simulink model "modelLiniarizat"  (R2022b)
settings: Solver=VariableStepAuto  StartTime=0.0  StopTime=50.0  RelTol=1e-3
values from neighbouring files (symbols this model uses):
  sys = ss(A_lin, B_lin, C_lin, D_lin)    [NeleptcuDanielAndrei.m]
undefined symbols (not defined in the file or in its folder): par, ustar8, xstar8, ystar8
settings Model: Creator=zuch3e  LastModifiedBy=zuch3e
settings DataIOCC: ReturnWorkspaceOutputs=off

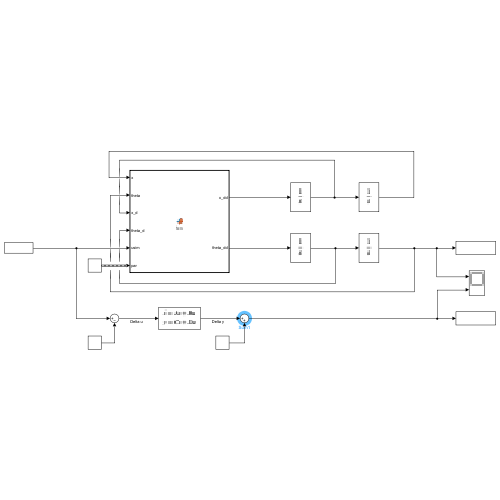
[thumbnail: Simulink's stored preview of the top-level diagram]
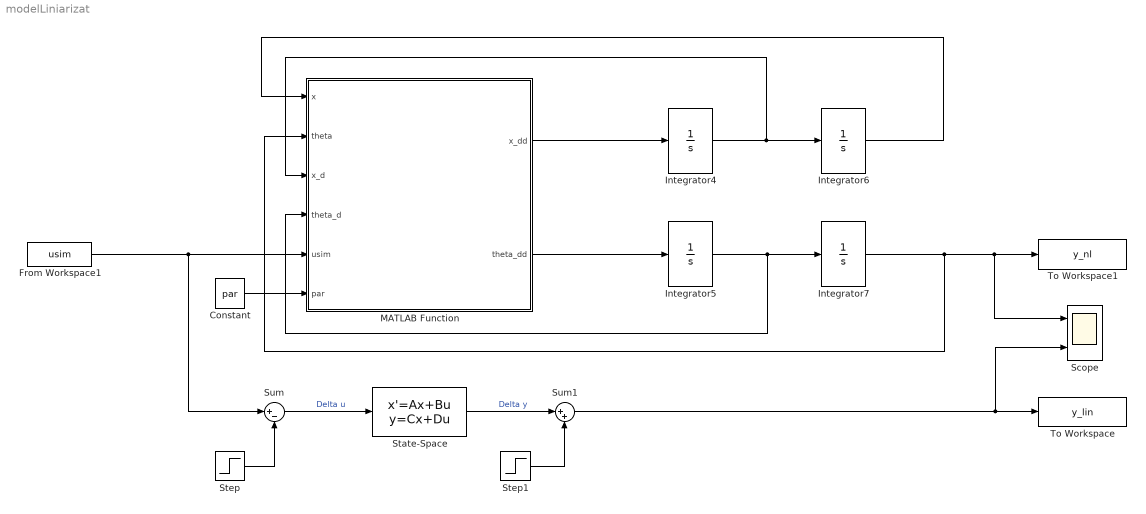
== system modelLiniarizat ==
  Constant : Constant  Value=par  OutDataTypeStr=Bus: par_bus
  From Workspace1 : FromWorkspace  VariableName=usim
  Integrator{4..7} (4 alike) : Integrator
  MATLAB Function : MATLAB Function  TreatAsAtomicUnit=on
  Scope : Scope  NumInputPorts=2
  State-Space : StateSpace  A=sys.A  B=sys.B  C=sys.C  D=sys.D  InitialCondition=-xstar8  ParameterTunability=Unconstrained
  Step : Step  After=ustar8  SampleTime=0
  Step1 : Step  After=ystar8  SampleTime=0
  Sum : Sum  Inputs=|+-
  Sum1 : Sum  Inputs=|++
  To Workspace : ToWorkspace  VariableName=y_lin  SaveFormat=Timeseries  SampleTime=-1
  To Workspace1 : ToWorkspace  VariableName=y_nl  SaveFormat=Timeseries  SampleTime=-1
  wires:
  Constant/1 -> MATLAB Function/6(par)
  Integrator7/1 -> MATLAB Function/2(theta), To Workspace1/1, Scope/1
  MATLAB Function/2(theta_dd) -> Integrator5/1
  Integrator5/1 -> MATLAB Function/4(theta_d), Integrator7/1
  Integrator6/1 -> MATLAB Function/1(x)
  MATLAB Function/1(x_dd) -> Integrator4/1
  Integrator4/1 -> MATLAB Function/3(x_d), Integrator6/1
  From Workspace1/1 -> MATLAB Function/5(usim), Sum/1
  Sum/1 -> State-Space/1  "Delta u"
  Step/1 -> Sum/2
  State-Space/1 -> Sum1/1  "Delta y"
  Step1/1 -> Sum1/2
  Sum1/1 -> Scope/2, To Workspace/1

== matlab function modelLiniarizat/MATLAB Function ==
  data: x input; x_dd output; theta input; x_d input; theta_d input; usim input; par input; theta_dd output
function [x_dd, theta_dd] = fcn(x,theta,x_d,theta_d,usim, par)
x_dd = ((par.l0 + x) * (theta_d^2)) - (par.k*x)/par.m + par.g*cos(theta) - par.zeta*x_d;
theta_dd = ((-1)*par.g*sin(theta))/(par.l0 + x) - (2*x_d*theta_d)/(par.l0 + x) - par.zeta*theta_d + usim/(par.m*((par.l0 + x)^2));
end
